simulink model "fadec_model"  (R2025b)
settings: Solver=FixedStepDiscrete  StartTime=0.0  StopTime=15  FixedStep=0.02  RelTol=1e-3
libraries: simulink x2
settings DataIOCC: InspectSignalLogs=on

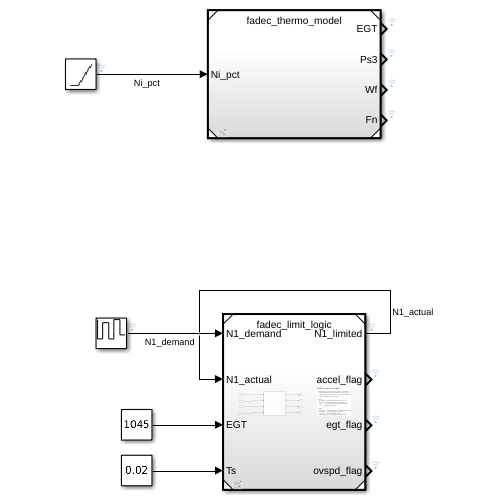
[thumbnail: Simulink's stored preview of the top-level diagram]
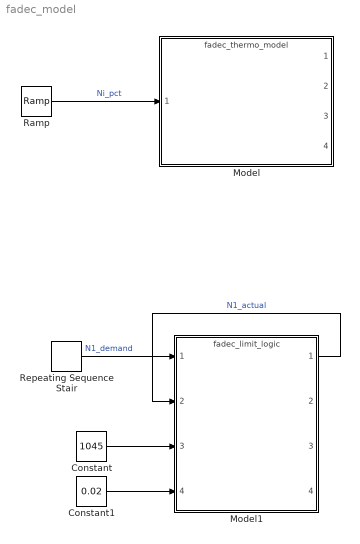
== system fadec_model ==
  Constant : Constant  Value=1045
  Constant1 : Constant  Value=0.02
  Model : ModelReference  ModelNameDialog=fadec_thermo_model.slx  SimulationMode=Normal  ModelReferenceVersion=1.13
  Model1 : ModelReference  ModelNameDialog=fadec_limit_logic.slx  SimulationMode=Normal  ModelReferenceVersion=1.4
  Ramp : simulink/Sources/Ramp  slope=10  start=0  InitialOutput=0  VectorParams1D=off
  Repeating Sequence Stair : simulink/Sources/Repeating Sequence Stair  OutValues=[19 95 19 110 40].'  tsamp=[5 3]  OutMin=[]  OutMax=[]  OutDataTypeStr=double  OutputDataTypeScalingMode=double  OutDataType=fixdt(0,8)  ConRadixGroup=Best Precision: Vector-wise  OutScaling=2^-12
  wires:
  Ramp/1 -> Model/1  "Ni_pct"
  Repeating Sequence Stair/1 -> Model1/1  "N1_demand"
  Model1/1 -> Model1/2  "N1_actual"
  Constant/1 -> Model1/3
  Constant1/1 -> Model1/4
